simulink model "control_model"  (R2023b)
settings: Solver=FixedStepAuto  StartTime=0.0  StopTime=18500  FixedStep=1  RelTol=1e-3
undefined symbols (not defined in the file or in its folder): t_step
settings Model: Creator=20181234  LastModifiedBy=20181234

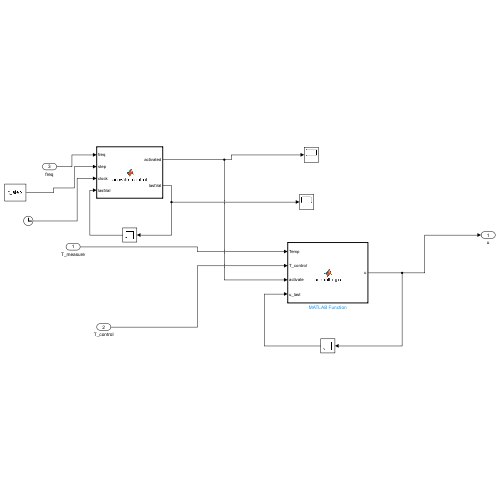
[thumbnail: Simulink's stored preview of the top-level diagram]
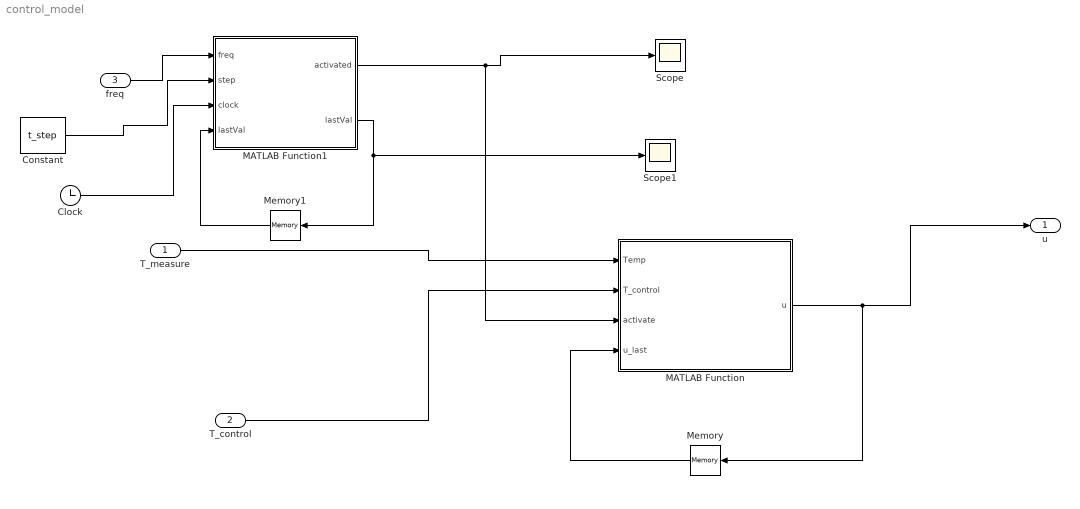
== system control_model ==
  T_measure : Inport
  T_control : Inport  Port=2
  freq : Inport  Port=3
  Clock : Clock
  Constant : Constant  Value=t_step
  MATLAB Function : MATLAB Function  TreatAsAtomicUnit=on
  MATLAB Function1 : MATLAB Function  TreatAsAtomicUnit=on
  Memory : Memory  LinearizeAsDelay=on
  Memory1 : Memory
  Scope : Scope
  Scope1 : Scope
  u : Outport
  wires:
  freq/1 -> MATLAB Function1/1(freq)
  MATLAB Function1/1(activated) -> MATLAB Function/3(activate), Scope/1
  Clock/1 -> MATLAB Function1/3(clock)
  Memory1/1 -> MATLAB Function1/4("lastVal ")
  MATLAB Function1/2(lastVal) -> Memory1/1, Scope1/1
  MATLAB Function/1(u) -> Memory/1, u/1
  Memory/1 -> MATLAB Function/4(u_last)
  Constant/1 -> MATLAB Function1/2(step)
  T_control/1 -> MATLAB Function/2(T_control)
  T_measure/1 -> MATLAB Function/1(Temp)

== matlab function control_model/MATLAB Function ==
  data: Temp input; u output; T_control input; activate input; u_last input
function u = controlLogic(Temp, T_control, activate, u_last)

if activate == true

    if Temp>= T_control
        u = 1;
    else
        u=0;
    end
else
    u= u_last;
end

== matlab function control_model/MATLAB Function1 ==
  data: freq input; activated output; step input; clock input; lastVal output; lastVal input
function [activated, lastVal]= activate_control(freq, step, clock, lastVal)



if clock == 0 || lastVal <= 0
    activated  = true;
    lastVal = freq;
else
    %lastVal = lastVal-step;
    activated = false;
end

lastVal = lastVal-step;
